simulink library "sun_estimation_lib"  (R2016a)
settings: Solver=ode45  StartTime=0.0  StopTime=86400  RelTol=1e-3
settings Model: Creator=Taylor  LastModifiedBy=bbarz_000
settings DataIOCC: LimitDataPoints=on
settings DebuggingCC: AllowSymbolicDim=off

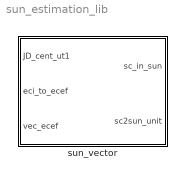
== system sun_estimation_lib ==
  sun_vector : Subsystem

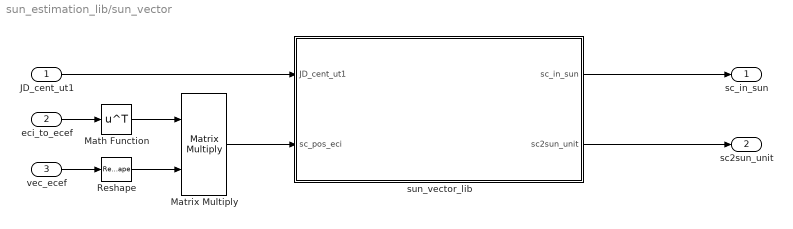
== system sun_estimation_lib/sun_vector ==
  JD_cent_ut1 : Inport
  eci_to_ecef : Inport  Port=2
  vec_ecef : Inport  Port=3
  Math Function : Math  Operator=transpose  SaturateOnIntegerOverflow=on
  Matrix Multiply : Product  Multiplication=Matrix(*)
  Reshape : Reshape  OutputDimensionality=Column vector (2-D)
  sun_vector_lib : Subsystem
  sc_in_sun : Outport
  sc2sun_unit : Outport  Port=2
  wires:
  JD_cent_ut1/1 -> sun_vector_lib/1(JD_cent_ut1)
  sun_vector_lib/1(sc_in_sun) -> sc_in_sun/1
  Matrix Multiply/1 -> sun_vector_lib/2(sc_pos_eci)
  eci_to_ecef/1 -> Math Function/1
  vec_ecef/1 -> Reshape/1
  Reshape/1 -> Matrix Multiply/2
  Math Function/1 -> Matrix Multiply/1
  sun_vector_lib/2(sc2sun_unit) -> sc2sun_unit/1

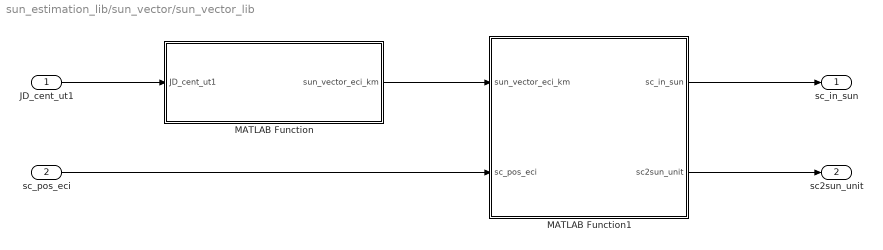
== system sun_estimation_lib/sun_vector/sun_vector_lib ==
  JD_cent_ut1 : Inport
  sc_pos_eci : Inport  Port=2
  MATLAB Function : MATLAB Function  TreatAsAtomicUnit=on
  MATLAB Function1 : MATLAB Function  TreatAsAtomicUnit=on
  sc_in_sun : Outport
  sc2sun_unit : Outport  Port=2
  wires:
  JD_cent_ut1/1 -> MATLAB Function/1(JD_cent_ut1)
  MATLAB Function/1(sun_vector_eci_km) -> MATLAB Function1/1(sun_vector_eci_km)
  sc_pos_eci/1 -> MATLAB Function1/2(sc_pos_eci)
  MATLAB Function1/2(sc2sun_unit) -> sc2sun_unit/1
  MATLAB Function1/1(sc_in_sun) -> sc_in_sun/1

== matlab function sun_estimation_lib/sun_vector/sun_vector_lib/MATLAB Function1 ==
  data: sun_vector_eci_km input; sc_in_sun output; sc2sun_unit output; sc_pos_eci input
function [sc_in_sun,sc2sun_unit] = sc_in_sun(sun_vector_eci_km,sc_pos_eci)

% Constants
M2KM        = 1000;
ECCE2       = 0.006694385000;
RE          = 6378.137;
TRUE        = 1;
FALSE       = 0;
% -----

% Convert to sc position vector to km if necessary
sc_pos_eci_km   = sc_pos_eci;
%-----

% Main Function
LOS     = FALSE;

sun_vector_eci_km(3)    = sun_vector_eci_km(3)/(sqrt(1 - ECCE2));
sc_pos_eci_km(3)        = sc_pos_eci_km(3)/(sqrt(1 - ECCE2));

sun_vec     = sun_vector_eci_km;
sc_vec      = sc_pos_eci_km;

sc2sun_unit  = (sun_vec - sc_vec)/norm(sun_vec - sc_vec);

% Determine if the sc is in the light or shadow
%   Call vector 1 the sun, vector 2 the sc

mag1    = norm(sun_vec);
mag2    = norm(sc_vec);

mag1_sq     = mag1*mag1;
mag2_sq     = mag2*mag2;

sun_sc_dot  = dot(sun_vec,sc_vec);

% Find t_min
t_min_num   = mag1_sq - sun_sc_dot;
t_min_den   = mag1_sq + mag2_sq - 2*sun_sc_dot;

if ( t_min_den < 0.0001  )
    t_min= 0.0;
else
    t_min = ( t_min_num ) / ( t_min_den );
end

c_t_min_sq  = ((1-t_min)*mag1_sq + sun_sc_dot*t_min)/RE^2;

% Check LoS
if t_min < 0 || t_min > 1
    LOS     = TRUE;
elseif c_t_min_sq >= 1
    LOS     = FALSE;
end

sc_in_sun   = LOS;

== matlab function sun_estimation_lib/sun_vector/sun_vector_lib/MATLAB Function ==
  data: JD_cent_ut1 input; sun_vector_eci_km output
function sun_vector_eci_km = sun_vector(JD_cent_ut1)

% Constants
AU2KM  = 149597870.700; 
DEG2RAD     = pi/180.0;
% -----

% Convert to Julian Centuries since J2000
% JD_cent_ut1     = (JD_ut1 - 2451545)/36525;

% Mean longitude in a mean-equator of date frame
mean_long_sun  = rem(280.460 + 36000.771*JD_cent_ut1,360); % [deg]

% Mean anomaly for the sun. Low precision formula since we're approximating
% T_TDB with T_UT1.
mean_anom_sun   = rem(357.5291092 + 35999.05034*JD_cent_ut1,360); %[deg]
mean_anom_sun_rad   = DEG2RAD*mean_anom_sun;

% Make sure we're \in [0,2pi]
if ( mean_anom_sun_rad < 0.0  )
    mean_anom_sun_rad = 2*pi + mean_anom_sun_rad;
end

% Approximate the ecliptic longitude of the sun
long_eclp       = mean_long_sun + 1.914666471*sin(mean_anom_sun_rad) + ...
                    0.019994643*sin(2*mean_anom_sun_rad); %[deg]
long_eclp_rad   = rem(DEG2RAD*long_eclp,360); % [rad]            
       
% Assume the ecliptic latitude is zero
lat_eclp     = 0; %[deg]

% Approximate the obliquity of the ecliptic using
oblq        = 23.439291 - 0.0130042*JD_cent_ut1;
oblq_rad    = DEG2RAD*oblq;

% Find the distance in AU from E to S
r           =  1.000140612 - 0.016708617*cos(mean_anom_sun_rad) - ...
                    0.000139589*cos(2*mean_anom_sun_rad);

x_MOD_km    = r*cos(long_eclp_rad)*AU2KM;
y_MOD_km    = r*cos(oblq_rad)*sin(long_eclp_rad)*AU2KM;
z_MOD_km    = r*sin(oblq_rad)*sin(long_eclp_rad)*AU2KM;

sun_vector_mod_km = [x_MOD_km; y_MOD_km; z_MOD_km];

% Convert to ECI (mean-equator-mean-equinox) frame 

sun_vector_eci_km   = mod2eci(sun_vector_mod_km,JD_cent_ut1);

end

function vec_eci = mod2eci(vec_mod,JD_cent_ut1)

[prec,psia,wa,ea,xa] = precess ( JD_cent_ut1 );

vec_eci = prec*vec_mod;

end

function [prec,psia,wa,ea,xa] = precess ( ttt )

        
        % " to rad
        convrt = pi / (180.0*3600.0);

          % ------------------ iau 03 precession angles -------------------
            oblo =  84381.406; % "
            psia =  (((( -0.0000000951 * ttt + 0.000132851 ) * ttt - 0.00114045 ) * ttt - 1.0790069 ) * ttt + 5038.481507 ) * ttt; % "
            wa   =  ((((  0.0000003337 * ttt - 0.000000467 ) * ttt - 0.00772503 ) * ttt + 0.0512623 ) * ttt -    0.025754 ) * ttt + oblo;
            ea   =  (((( -0.0000000434 * ttt - 0.000000576 ) * ttt + 0.00200340 ) * ttt - 0.0001831 ) * ttt -   46.836769 ) * ttt + oblo;
            xa   =  (((( - 0.0000000560 * ttt + 0.000170663 ) * ttt - 0.00121197 ) * ttt - 2.3814292 ) * ttt +   10.556403 ) * ttt;

            zeta =  (((( - 0.0000003173 * ttt - 0.000005971 ) * ttt + 0.01801828 ) * ttt + 0.2988499 ) * ttt + 2306.083227 ) * ttt + 2.650545; % "
            theta=  (((( - 0.0000001274 * ttt - 0.000007089 ) * ttt - 0.04182264 ) * ttt - 0.4294934 ) * ttt + 2004.191903 ) * ttt;
            z    =  ((((   0.0000002904 * ttt - 0.000028596 ) * ttt + 0.01826837 ) * ttt + 1.0927348 ) * ttt + 2306.077181 ) * ttt - 2.650545;
        
        % convert all units to rad
        psia = psia  * convrt; % rad
        wa   = wa    * convrt;
        ea   = ea    * convrt;
        xa   = xa    * convrt;

            oblo = oblo * convrt; % " to rad
            a4  = rot3mat(-xa);
            a5  = rot1mat(wa);
            a6  = rot3mat(psia);
            a7  = rot1mat(-oblo);
            prec = a7*a6*a5*a4;
        
end % precess

function DCMx = rot1mat(x_rad)

s   = sin( x_rad );
c   = cos( x_rad );

DCMx    = [ 1   0   0
            0   c   s;
            0  -s   c ];

end

function DCMz   = rot3mat(z_rad)

s   = sin( z_rad );
c   = cos( z_rad );

DCMz    = [ c   s   0;
           -s   c   0;
            0   0   1 ];

end
